simulink subsystem "Environment_Model"  (R2020b)
settings: Solver=VariableStepAuto  StartTime=0.0  StopTime=10.0  RelTol=1e-3
libraries: aerolibconvert2 x1
settings Model: Creator=Fatih  LastModifiedBy=Fatih

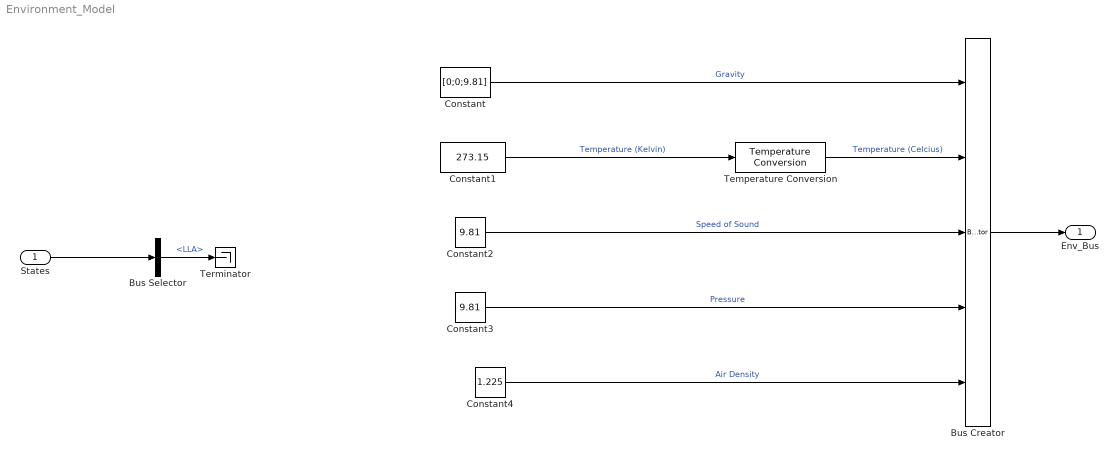
== system Environment_Model ==
  States : Inport
  Bus Creator : BusCreator  Inputs=5
  Bus Selector : BusSelector  OutputSignals=LLA
  Constant : Constant  Value=[0;0;9.81]
  Constant1 : Constant  Value=273.15
  Constant2 : Constant  Value=9.81
  Constant3 : Constant  Value=9.81
  Constant4 : Constant  Value=1.225
  Temperature Conversion : aerolibconvert2/Temperature Conversion  IU=K  OU=C
      settings: SourceProductBaseCode=AE
  Terminator : Terminator
  Env_Bus : Outport
  wires:
  Constant/1 -> Bus Creator/1  "Gravity"
  Constant1/1 -> Temperature Conversion/1  "Temperature (Kelvin)"
  Constant2/1 -> Bus Creator/3  "Speed of Sound"
  Constant3/1 -> Bus Creator/4  "Pressure"
  Constant4/1 -> Bus Creator/5  "Air Density"
  Temperature Conversion/1 -> Bus Creator/2  "Temperature (Celcius)"
  Bus Creator/1 -> Env_Bus/1
  States/1 -> Bus Selector/1
  Bus Selector/1 -> Terminator/1  "<LLA>"
